simulink model "lab4"  (R2021b)
settings: Solver=VariableStepAuto  StartTime=0.0  StopTime=15  MaxStep=0.001  RelTol=1e-3
settings Model: PacingRate=0.500000  Creator=asr77  LastModifiedBy=asr77

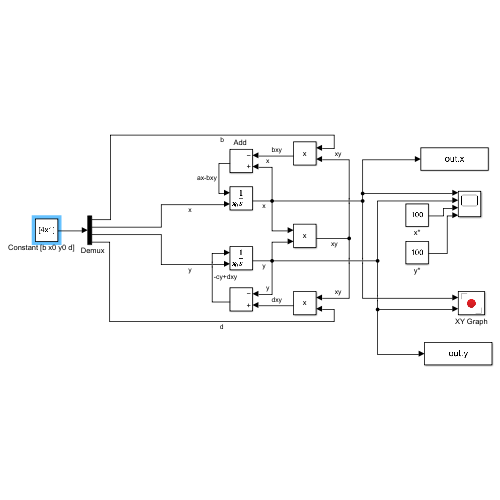
[thumbnail: Simulink's stored preview of the top-level diagram]
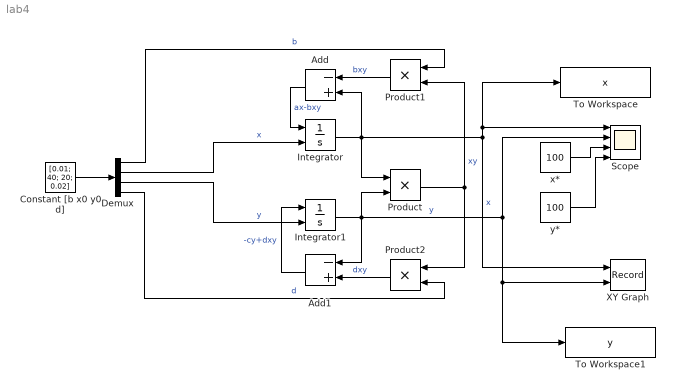
== system lab4 ==
  "   Demux" : Demux
  "Add " : Sum  Inputs=-+
  Add1 : Sum  Inputs=-+
  "Constant [b x0 y0 d]     " : Constant  Value=[0.01; 40; 20; 0.02]
  Integrator : Integrator  InitialConditionSource=external
  Integrator1 : Integrator  InitialConditionSource=external
  Product : Product
  Product1 : Product
  Product2 : Product
  Scope : Scope  NumInputPorts=4
  To Workspace : ToWorkspace  VariableName=x  SaveFormat=Timeseries  SampleTime=-1
  To Workspace1 : ToWorkspace  VariableName=y  SaveFormat=Timeseries  SampleTime=-1
  XY Graph : Record  FileSettingsInternal="{\"entries\":[{\"content\":{\"excelSettings\":{\"content\":{},\"type\":\"Streamout.ExcelSettings\"}},\"type\":\"Streamout.FileSettingStorage\",\"uuid\":\"890cfd2d-f087-4fc4-b885-9de09324d6f0\"}],\"packageUris\":[\"http://schema.mathworks.com/mf0/streamout_blocks/R2020a\"],\"version\":\"1.0\"}"  Layout=[1 1]  SignalsInternal="{\"entries\":[{\"content\":{\"signals\":[{\"content\":{\"blockPath\":[\"lab4/XY Graph\"],\"channel\":[],\"dimensions\":[1],\"domain\":\"lab4/XY Graph\",\"lineColor\":\"#a2142f\",\"plots\":[1],\"port\":1,\"sid\":[\"\"],\"signalID\":192,\"signalName\":\"x\"},\"type\":\"RecordBlkView.Signal\",\"uuid\":\"140f5371-95d5-4027-a414-49ca6ce7089f\"},{\"content\":{\"blockPath\":[\"lab4/XY Graph\"],\"channel\":[],\"dimensions\":[1],\"domain\":\"lab4/XY Graph\",\"lineColor\":\"#139fff\",\"plots\":[1],\"port\":2,\"sid\":[\"\"],\"signalID\":196,\"signalName\":\"y\"},\"type\":\"RecordBlkView.Signal\",\"uuid\":\"500c7cf5-0353-4722-ace3-cfe524afd4fe\"}]},\"type\":\"RecordBlkView.InputSignals\",\"uuid\":\"37746088-3099-48c8-8705-795e92ca1e4e\"}],\"packageUris\":[\"http://schema.mathworks.com/mf0/streamout_blocks/R2020a\"],\"version\":\"1.0\"}"  VisualizationBindings="{\"xyplotplugin\":{\"info\":[{\"series\":[{\"bindingParametersList\":[{\"parameter\":\"X-Axis\",\"signalID\":192,\"signalName\":\"x\"},{\"parameter\":\"Y-Axis\",\"signalID\":196,\"signalName\":\"y\"}],\"seriesID\":53242}],\"subplotID\":1}]}}"  CompatibilityTag=XY
  x* : Constant  Value=100
  y* : Constant  Value=100
  wires:
  "Constant [b x0 y0 d]     "/1 -> "   Demux"/1
  Product1/1 -> "Add "/1  "bxy"
  Product2/1 -> Add1/2  "dxy"
  "   Demux"/2 -> Integrator/2  "x"
  "   Demux"/3 -> Integrator1/2  "y"
  Add1/1 -> Integrator1/1  "-cy+dxy"
  "Add "/1 -> Integrator/1  "ax-bxy"
  "   Demux"/1 -> Product1/1  "b"
  "   Demux"/4 -> Product2/2  "d"
  Integrator1/1 -> Add1/1, Product/2, To Workspace1/1, XY Graph/2, Scope/2  "y"
  Integrator/1 -> "Add "/2, Product/1, Scope/1, To Workspace/1, XY Graph/1  "x"
  Product/1 -> Product1/2, Product2/1  "xy"
  x*/1 -> Scope/3
  y*/1 -> Scope/4
